simulink model "Double_Pendulum_Euler_Lagrange_with_damper"  (R2021b)
settings: Solver=VariableStepAuto  StartTime=0.0  StopTime=40  RelTol=1e-3
settings Model: Creator=Spino.shop  LastModifiedBy=Spino.shop

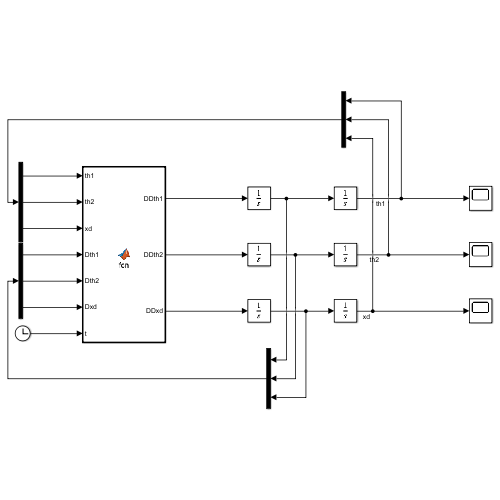
[thumbnail: Simulink's stored preview of the top-level diagram]
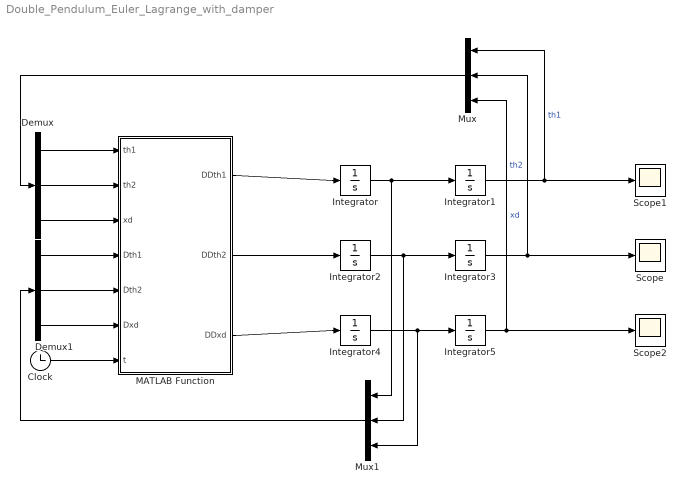
== system Double_Pendulum_Euler_Lagrange_with_damper ==
  Clock : Clock
  Demux : Demux  Outputs=3
  Demux1 : Demux  Outputs=3
  Integrator{,1..5} (6 alike) : Integrator
  MATLAB Function : MATLAB Function  TreatAsAtomicUnit=on
  Mux : Mux  Inputs=3
  Mux1 : Mux  Inputs=3
  Scope : Scope
  Scope1 : Scope
  Scope2 : Scope
  wires:
  Integrator/1 -> Mux1/1, Integrator1/1
  Integrator2/1 -> Mux1/2, Integrator3/1
  Integrator4/1 -> Mux1/3, Integrator5/1
  MATLAB Function/3(DDxd) -> Integrator4/1
  MATLAB Function/2(DDth2) -> Integrator2/1
  MATLAB Function/1(DDth1) -> Integrator/1
  Integrator1/1 -> Scope1/1, Mux/1  "th1"
  Integrator3/1 -> Scope/1, Mux/2  "th2"
  Clock/1 -> MATLAB Function/7(t)
  Integrator5/1 -> Scope2/1, Mux/3  "xd"
  Demux/3 -> MATLAB Function/3(xd)
  Demux/1 -> MATLAB Function/1(th1)
  Demux/2 -> MATLAB Function/2(th2)
  Mux/1 -> Demux/1
  Mux1/1 -> Demux1/1
  Demux1/1 -> MATLAB Function/4(Dth1)
  Demux1/2 -> MATLAB Function/5(Dth2)
  Demux1/3 -> MATLAB Function/6(Dxd)

== matlab function Double_Pendulum_Euler_Lagrange_with_damper/MATLAB Function ==
  data: th1 input; th2 input; xd input; Dth1 input; Dth2 input; Dxd input; DDth1 output; DDth2 output; DDxd output; t input
function [DDth1, DDth2, DDxd] = fcn(th1, th2, xd, Dth1, Dth2, Dxd, t)

Y = zeros(6,1);
Y(1) = xd;
Y(2) = Dxd;
Y(3) = th1;
Y(4) = Dth1;
Y(5) = th2;
Y(6) = Dth2;

DDxd = -(cos(Y(3) - Y(5))^2*Y(1) - sin(t) + cos(Y(3) - Y(5))^2*Y(2) - cos(Y(5))*cos(Y(3) - Y(5)) ...
        + sin(Y(3) - Y(5))*Y(6)^2 - sin(Y(3))*Y(1) + cos(Y(3))*cos(Y(3) - Y(5))^2 ...
        - cos(Y(3) - Y(5))*Y(6) - 3*Y(1) - 3*Y(2) + Y(4) + cos(Y(3) - Y(5))*cos(t) ...
        + cos(Y(3) - Y(5))*sin(Y(3) - Y(5))*Y(4)^2)/(cos(Y(3) - Y(5))^2 - 2);

DDth1 = -(sin(t) - 2*cos(Y(3)) + cos(Y(5))*cos(Y(3) - Y(5)) - sin(Y(3) - Y(5))*Y(6)^2 ...
    + sin(Y(3))*Y(1) + cos(Y(3) - Y(5))*Y(6) + Y(1) + Y(2) - Y(4) - cos(Y(3) - Y(5))*cos(t) ...
    - cos(Y(3) - Y(5))*sin(Y(3) - Y(5))*Y(4)^2)/(cos(Y(3) - Y(5))^2 - 2);

DDth2 = (2*cos(Y(5)) - 2*cos(t) - 2*cos(Y(3))*cos(Y(3) - Y(5)) - 2*sin(Y(3) - Y(5))*Y(4)^2 ...
    + cos(Y(3) - Y(5))*Y(1) + cos(Y(3) - Y(5))*Y(2) - cos(Y(3) - Y(5))*Y(4) + 2*Y(6) ...
    + cos(Y(3) - Y(5))*sin(t) - cos(Y(3) - Y(5))*sin(Y(3) - Y(5))*Y(6)^2 ...
    + sin(Y(3))*cos(Y(3) - Y(5))*Y(1))/(cos(Y(3) - Y(5))^2 - 2);
